simulink model "agreement"  (R2021b)
settings: Solver=FixedStepAuto  StartTime=0.0  StopTime=10.0  FixedStep=0.20000000000000001  RelTol=1e-3
undefined symbols (not defined in the file): sldvsubsys
libraries: sldvlib x7
settings Model: Creator=marco  LastModifiedBy=angelo
settings DataIOCC: SaveOutput=off  DSMLogging=off  SaveTime=off  SignalLoggingName=logsout_Validator
settings DebuggingCC: InheritedTsInSrcMsg=none
settings ModelReferenceCC: UpdateModelReferenceTargets=IfOutOfDate
settings ConfigComp: CovEnable=on  RecordCoverage=on  CovSaveName=coveragedata  CovMetricSettings=owe  CovEnableCumulative=off  CovSaveSingleToWorkspaceVar=on  CovOutputDir=sldv_covoutput/agreement  CovModelRefEnable=on  CovSFcnEnable=off  DVMode=PropertyProving  DVMaxProcessTime=21600  DVTestSuiteOptimization=Auto  DVDetectOutOfBounds=on  DVModelReferenceHarness=on

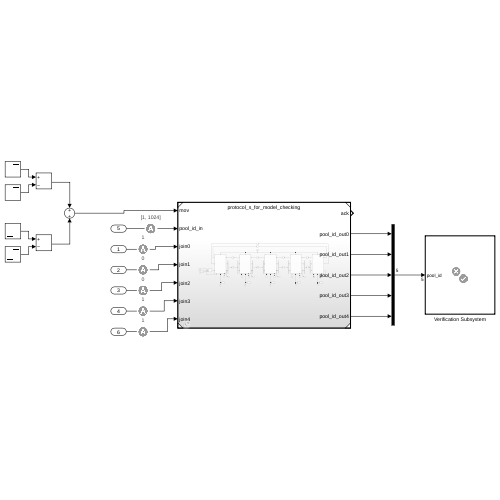
[thumbnail: Simulink's stored preview of the top-level diagram]
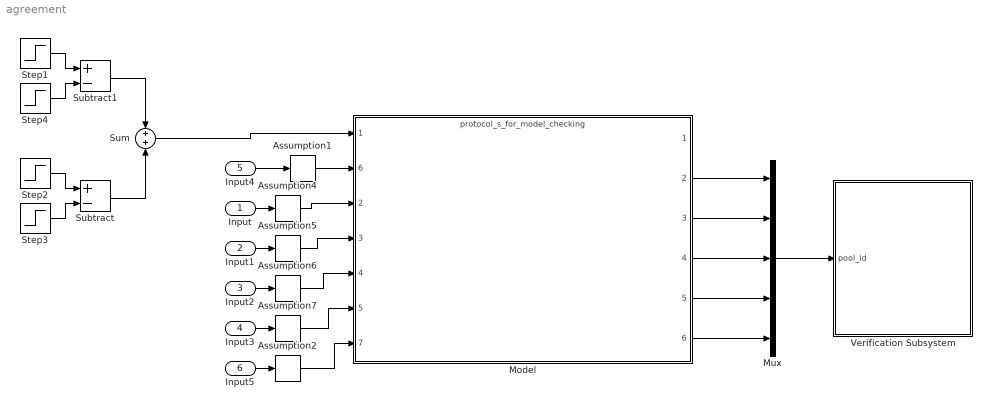
== system agreement ==
  Input : Inport
  Input1 : Inport  Port=2
  Input2 : Inport  Port=3
  Input3 : Inport  Port=4
  Input4 : Inport  Port=5
  Input5 : Inport  Port=6
  Assumption1 : sldvlib/Objectives and Constraints/Assumption  enabled=on  customAVTBlockType=Assumption  intervals=[1, 1024]  initial=off  dispValues=on  outEnabled=on
      settings: AttributesFormatString=%<intervals>  SourceProductBaseCode=SL
  Assumption2 : sldvlib/Objectives and Constraints/Assumption  enabled=on  customAVTBlockType=Assumption  intervals=1  initial=off  dispValues=on  outEnabled=on
      settings: AttributesFormatString=%<intervals>  SourceProductBaseCode=SL
  Assumption4 : sldvlib/Objectives and Constraints/Assumption  enabled=on  customAVTBlockType=Assumption  intervals=1  initial=off  dispValues=on  outEnabled=on
      settings: AttributesFormatString=%<intervals>  SourceProductBaseCode=SL
  Assumption5 : sldvlib/Objectives and Constraints/Assumption  enabled=on  customAVTBlockType=Assumption  intervals=0  initial=off  dispValues=on  outEnabled=on
      settings: AttributesFormatString=%<intervals>  SourceProductBaseCode=SL
  Assumption6 : sldvlib/Objectives and Constraints/Assumption  enabled=on  customAVTBlockType=Assumption  intervals=0  initial=off  dispValues=on  outEnabled=on
      settings: AttributesFormatString=%<intervals>  SourceProductBaseCode=SL
  Assumption7 : sldvlib/Objectives and Constraints/Assumption  enabled=on  customAVTBlockType=Assumption  intervals=1  initial=off  dispValues=on  outEnabled=on
      settings: AttributesFormatString=%<intervals>  SourceProductBaseCode=SL
  Model : ModelReference  ModelNameDialog=protocol_s_for_model_checking.slx  SimulationMode=Normal  ModelReferenceVersion=1.126
      settings: PortSchema="{\"entries\":[{\"content\":{\"sides\":[{\"content\":{\"connectorIds\":[\"In1\",\"In6\",\"In2\",\"In3\",\"In4\",\"In5\",\"In7\"]},\"type\":\"ConnectorPlacement.EquallySpacedRectSide\",\"uuid\":\"2cc34edd-a176-40cb-b6fa-8cbf6e460119\"},{\"content\":{\"connectorIds\":[\"Out1\",\"Out2\",\"Out3\",\"Out4\",\"Out5\",\"Out6\"],\"side\":\"RIGHT\"},\"type\":\"ConnectorPlacement.EquallySpacedRectSide\",\"uuid\":\"b9fb4b35-80b7-4954-be48-a4c9e0c81b3a\"},{\"content\":{\"connectorIds\":[],\"side\":\"TOP\"},\"type\":\"ConnectorPlacement.EquallySpacedRectSide\",\"uuid\":\"9d4ba344-f407-4b95-9191-bce6cbc03920\"}]},\"type\":\"ConnectorPlacement.EquallySpacedConnector\",\"uuid\":\"c770100c-051e-4872-aa3a-ba047be3662c\"}],\"packageUris\":[\"http://schema.mathworks.com/mf0/Connector/R2020b\"],\"version\":\"1.0\"}"
  Mux : Mux  Inputs=5
  Step1 : Step  Time=.2  SampleTime=.2
  Step2 : Step  SampleTime=.2
  Step3 : Step  Time=1.2  SampleTime=.2
  Step4 : Step  Time=.4  SampleTime=.2
  Subtract : Sum  Inputs=+-
  Subtract1 : Sum  Inputs=+-
  Sum : Sum
  Verification Subsystem : Subsystem  Tag=VerificationSubsystem  DisableCoverage=on  LoadFcn=sldvsubsys('check')  TreatAsAtomicUnit=on  SimViewingDevice=on  mask(VerificationSubsystem){}
      mask init:
      | sldvsubsys('maskInit');
      settings: CopyFcn=sldvsubsys('copy');  OpenFcn=open_system(gcb,'force');
      settings: PreSaveFcn=|
      | set_param(gcb,'SimViewingDevice','on');
      | sldvsubsys('check');
      mask Help: helpview(fullfile(docroot,'toolbox','sldv','sldv.map'),'verificationsubsystem')
      mask Display: image(imread('sldvicon_versubsys.png','BackGroundColor',[1 1 1]),'center');
  wires:
  Step2/1 -> Subtract/1
  Step3/1 -> Subtract/2
  Input1/1 -> Assumption5/1
  Input2/1 -> Assumption6/1
  Input/1 -> Assumption4/1
  Input3/1 -> Assumption7/1
  Assumption4/1 -> Model/2
  Assumption5/1 -> Model/3
  Assumption6/1 -> Model/4
  Assumption7/1 -> Model/5
  Mux/1 -> Verification Subsystem/1(pool_id)
  Step1/1 -> Subtract1/1
  Step4/1 -> Subtract1/2
  Subtract1/1 -> Sum/1
  Assumption1/1 -> Model/6
  Subtract/1 -> Sum/2
  Sum/1 -> Model/1
  Input4/1 -> Assumption1/1
  Model/2 -> Mux/1
  Model/3 -> Mux/2
  Model/4 -> Mux/3
  Model/5 -> Mux/4
  Assumption2/1 -> Model/7
  Input5/1 -> Assumption2/1
  Model/6 -> Mux/5

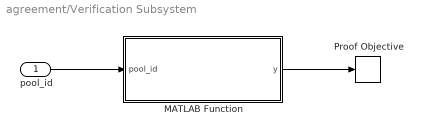
== system agreement/Verification Subsystem ==
  pool_id : Inport
  MATLAB Function : MATLAB Function  TreatAsAtomicUnit=on
  Proof Objective : sldvlib/Objectives and Constraints/Proof Objective  enabled=on  customAVTBlockType=Proof Objective  intervals=true  dispValues=on  outEnabled=off  enableStopSim=off
      settings: AttributesFormatString=%<intervals>  SourceProductBaseCode=SL
  wires:
  pool_id/1 -> MATLAB Function/1(pool_id)
  MATLAB Function/1(y) -> Proof Objective/1

== matlab function agreement/Verification Subsystem/MATLAB Function ==
  data: pool_id input; y output
function y = agreement(pool_id)
    y = all((pool_id == max(pool_id)) | (pool_id == 0));
end
